simulink model "TST_DYN_GRAV"  (R2017b)
settings: Solver=VariableStepAuto  StartTime=0.0  StopTime=30000  RelTol=1e-3
libraries: DYN_GRAV x1
settings Model: Creator=WilTravis  LastModifiedBy=Mahal

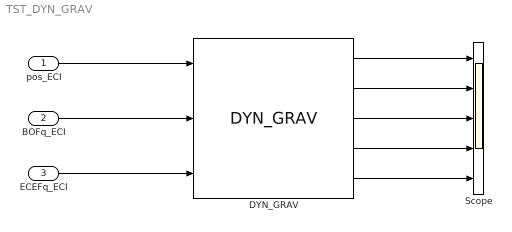
== system TST_DYN_GRAV ==
  pos_ECI : Inport
  BOFq_ECI : Inport  Port=2
  ECEFq_ECI : Inport  Port=3
  DYN_GRAV : DYN_GRAV/DYN_GRAV
  Scope : Scope  NumInputPorts=5
  wires:
  ECEFq_ECI/1 -> DYN_GRAV/3
  BOFq_ECI/1 -> DYN_GRAV/2
  pos_ECI/1 -> DYN_GRAV/1
  DYN_GRAV/1 -> Scope/1
  DYN_GRAV/2 -> Scope/2
  DYN_GRAV/3 -> Scope/3
  DYN_GRAV/4 -> Scope/4
  DYN_GRAV/5 -> Scope/5
